simulink model "plot_dynamic_3Drobot"  (R2021a)
settings: Solver=VariableStepAuto  StartTime=0.0  StopTime=100  FixedStep=10e-3  RelTol=1e-3  AbsTol=1e-3  EnableMultiTasking=on
undefined symbols (not defined in the file): C, H, L, L1, L2, L3, X, Y, Z
libraries: sm_lib x38, roblocks x20, nesl_utility x13, simulink x1
settings Model: Creator=Usuário  LastModifiedBy=Usuário
settings SolverCC: AutoScaleAbsTol=off  AlgebraicLoopSolver=TrustRegion
settings DataIOCC: LimitDataPoints=on  MaxDataPoints=10000
settings OptimizationCC: LifeSpan=inf
settings DebuggingCC: AllowSymbolicDim=off  SFUnexpectedBacktrackingDiag=warning  SFNoUnconditionalDefaultTransitionDiag=warning  SFExecutionAtInitializationDiag=none  SFMachineParentedDataDiag=warning  ArithmeticOperatorsInVariantConditions=warning
settings SFSimCC: SimUseLocalCustomCode=off  CustomCodeUndefinedFunction=UseInterfaceOnly
settings RTWCC: RTWUseLocalCustomCode=off
settings CodeAppCC: StateflowObjectComments=on
settings GRTTargetCC: TargetLangStandard=C89/C90 (ANSI)
settings ConfigComp: CovMetricSettings=dw  CovSaveCumulativeToWorkspaceVar=on  CovSaveSingleToWorkspaceVar=on  CovExternalEMLEnable=off  CovSFcnEnable=off
settings SimscapeCC: SimscapeLogType=all  SimscapeLogSimulationStatistics=on  SimscapeLogDataHistory=10000

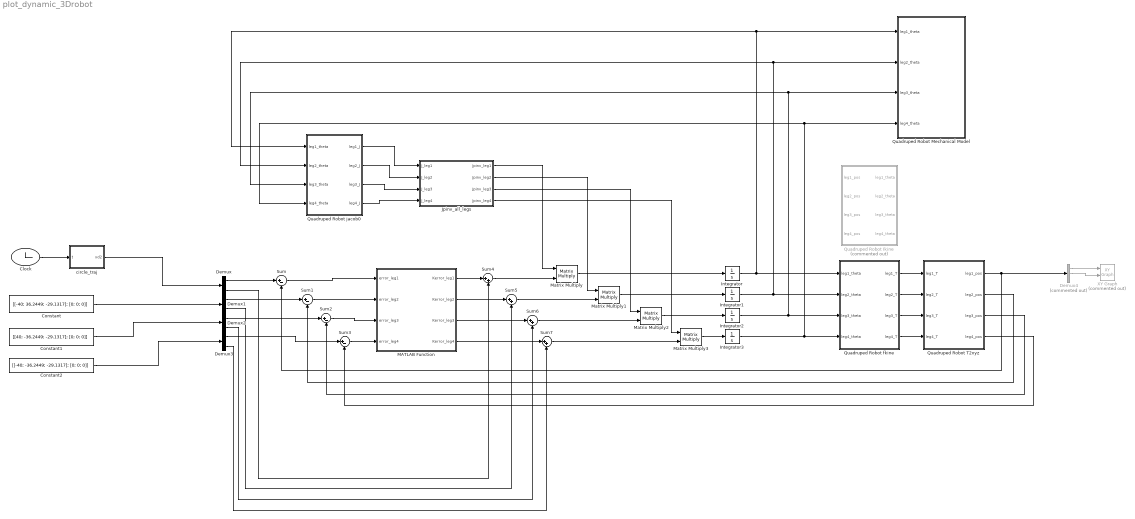
== system plot_dynamic_3Drobot ==
  Clock : Clock
  Constant : Constant  Value=[[-40; 36.2449; -29.1317]; [0; 0; 0]]
  Constant1 : Constant  Value=[[40; -36.2449; -29.1317]; [0; 0; 0]]
  Constant2 : Constant  Value=[[-40; -36.2449; -29.1317]; [0; 0; 0]]
  Demux{,1..3} (4 alike) : Demux  Outputs=2
  Demux4 : Demux  Commented=on  Outputs=3
  Integrator{,1..3} (4 alike) : Integrator
  Jpinv_all_legs : MATLAB Function  TreatAsAtomicUnit=on
  MATLAB Function : MATLAB Function  TreatAsAtomicUnit=on
  Matrix Multiply{,1..3} (4 alike) : Product  Multiplication=Matrix(*)
  Quadruped Robot Ikine : Subsystem  Commented=on
  Quadruped Robot Mechanical Model : Subsystem
  Quadruped Robot T2xyz : Subsystem
  Quadruped Robot fkine : Subsystem
  Quadruped Robot jacob0 : Subsystem
  Sum{,1..3} (4 alike) : Sum  Inputs=|+-
  Sum{4..7} (4 alike) : Sum  Inputs=|++
  XY Graph : simulink/Sinks/XY Graph  Commented=on  xmin=-100  xmax=100  ymin=-100  ymax=100  st=-1
  circle_traj : MATLAB Function  TreatAsAtomicUnit=on
  wires:
  Constant/1 -> Demux1/1
  Constant1/1 -> Demux2/1
  circle_traj/1(xd2) -> Demux/1
  Constant2/1 -> Demux3/1
  Clock/1 -> circle_traj/1(t)
  Quadruped Robot jacob0/1(leg1_J) -> Jpinv_all_legs/1(J_leg1)
  Quadruped Robot jacob0/2(leg2_J) -> Jpinv_all_legs/2(J_leg2)
  Quadruped Robot jacob0/3(leg3_J) -> Jpinv_all_legs/3(J_leg3)
  Quadruped Robot jacob0/4(leg4_J) -> Jpinv_all_legs/4(J_leg4)
  Demux/1 -> Sum/1
  Demux1/1 -> Sum1/1
  Demux2/1 -> Sum2/1
  Demux3/1 -> Sum3/1
  Sum/1 -> MATLAB Function/1(error_leg1)
  Sum1/1 -> MATLAB Function/2(error_leg2)
  Sum2/1 -> MATLAB Function/3(error_leg3)
  Sum3/1 -> MATLAB Function/4(error_leg4)
  MATLAB Function/1(Kerror_leg1) -> Sum4/1
  MATLAB Function/2(Kerror_leg2) -> Sum5/1
  MATLAB Function/3(Kerror_leg3) -> Sum6/1
  MATLAB Function/4(Kerror_leg4) -> Sum7/1
  Demux/2 -> Sum4/2
  Demux1/2 -> Sum5/2
  Demux2/2 -> Sum6/2
  Demux3/2 -> Sum7/2
  Sum4/1 -> Matrix Multiply/2
  Sum5/1 -> Matrix Multiply1/2
  Sum6/1 -> Matrix Multiply2/2
  Sum7/1 -> Matrix Multiply3/2
  Jpinv_all_legs/1(Jpinv_leg1) -> Matrix Multiply/1
  Jpinv_all_legs/2(Jpinv_leg2) -> Matrix Multiply1/1
  Jpinv_all_legs/3(Jpinv_leg3) -> Matrix Multiply2/1
  Jpinv_all_legs/4(Jpinv_leg4) -> Matrix Multiply3/1
  Matrix Multiply/1 -> Integrator/1
  Matrix Multiply1/1 -> Integrator1/1
  Matrix Multiply2/1 -> Integrator2/1
  Matrix Multiply3/1 -> Integrator3/1
  Integrator/1 -> Quadruped Robot fkine/1(leg1_theta), Quadruped Robot jacob0/1(leg1_theta), Quadruped Robot Mechanical Model/1(leg1_theta)
  Integrator1/1 -> Quadruped Robot fkine/2(leg2_theta), Quadruped Robot Mechanical Model/2(leg2_theta), Quadruped Robot jacob0/2(leg2_theta)
  Integrator2/1 -> Quadruped Robot fkine/3(leg3_theta), Quadruped Robot Mechanical Model/3(leg3_theta), Quadruped Robot jacob0/3(leg3_theta)
  Integrator3/1 -> Quadruped Robot fkine/4(leg4_theta), Quadruped Robot Mechanical Model/4(leg4_theta), Quadruped Robot jacob0/4(leg4_theta)
  Quadruped Robot fkine/1(leg1_T) -> Quadruped Robot T2xyz/1(leg1_T)
  Quadruped Robot fkine/2(leg2_T) -> Quadruped Robot T2xyz/2(leg2_T)
  Quadruped Robot fkine/3(leg3_T) -> Quadruped Robot T2xyz/3(leg3_T)
  Quadruped Robot fkine/4(leg4_T) -> Quadruped Robot T2xyz/4(leg4_T)
  Quadruped Robot T2xyz/1(leg1_pos) -> Demux4/1, Sum/2
  Quadruped Robot T2xyz/2(leg2_pos) -> Sum1/2
  Quadruped Robot T2xyz/3(leg3_pos) -> Sum2/2
  Quadruped Robot T2xyz/4(leg4_pos) -> Sum3/2
  Demux4/1 -> XY Graph/1
  Demux4/2 -> XY Graph/2

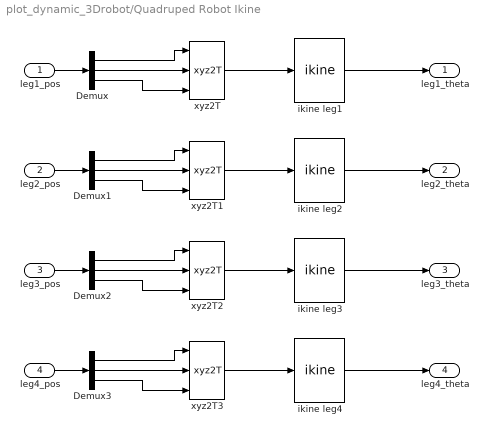
== system plot_dynamic_3Drobot/Quadruped Robot Ikine ==
  leg1_pos : Inport
  leg2_pos : Inport  Port=2
  leg3_pos : Inport  Port=3
  leg4_pos : Inport  Port=4
  Demux{,1..3} (4 alike) : Demux  Outputs=3
  ikine leg1 : roblocks/Arm/ikine  robot=leg1  q0=[0, 0, 0]  M=[1 1 1 0 0 0]  pinv=off  options={'ilimit', 10e4}
      link override ikine: MATLABFcn=robot.ikine(u, 'q0', q0, 'mask', M, opt{:})
  ikine leg2 : roblocks/Arm/ikine  robot=leg2  q0=[0, 0, 0]  M=[1 1 1 0 0 0]  pinv=off  options={'ilimit', 10e4}
      link override ikine: MATLABFcn=robot.ikine(u, 'q0', q0, 'mask', M, opt{:})
  ikine leg3 : roblocks/Arm/ikine  robot=leg3  q0=[0, 0, 0]  M=[1 1 1 0 0 0]  pinv=off  options={'ilimit', 10e4}
      link override ikine: MATLABFcn=robot.ikine(u, 'q0', q0, 'mask', M, opt{:})
  ikine leg4 : roblocks/Arm/ikine  robot=leg4  q0=[0, 0, 0]  M=[1 1 1 0 0 0]  pinv=off  options={'ilimit', 10e4}
      link override ikine: MATLABFcn=robot.ikine(u, 'q0', q0, 'mask', M, opt{:})
  xyz2T{,1..3} (4 alike) : roblocks/Toolbox/xyz2T
  leg1_theta : Outport
  leg2_theta : Outport  Port=2
  leg3_theta : Outport  Port=3
  leg4_theta : Outport  Port=4
  wires:
  xyz2T/1 -> ikine leg1/1
  leg1_pos/1 -> Demux/1
  Demux/1 -> xyz2T/1
  Demux/2 -> xyz2T/2
  Demux/3 -> xyz2T/3
  Demux1/2 -> xyz2T1/2
  Demux1/3 -> xyz2T1/3
  Demux1/1 -> xyz2T1/1
  leg2_pos/1 -> Demux1/1
  xyz2T1/1 -> ikine leg2/1
  Demux2/2 -> xyz2T2/2
  Demux2/3 -> xyz2T2/3
  Demux2/1 -> xyz2T2/1
  leg3_pos/1 -> Demux2/1
  xyz2T2/1 -> ikine leg3/1
  Demux3/2 -> xyz2T3/2
  Demux3/3 -> xyz2T3/3
  Demux3/1 -> xyz2T3/1
  leg4_pos/1 -> Demux3/1
  xyz2T3/1 -> ikine leg4/1
  ikine leg1/1 -> leg1_theta/1
  ikine leg2/1 -> leg2_theta/1
  ikine leg3/1 -> leg3_theta/1
  ikine leg4/1 -> leg4_theta/1

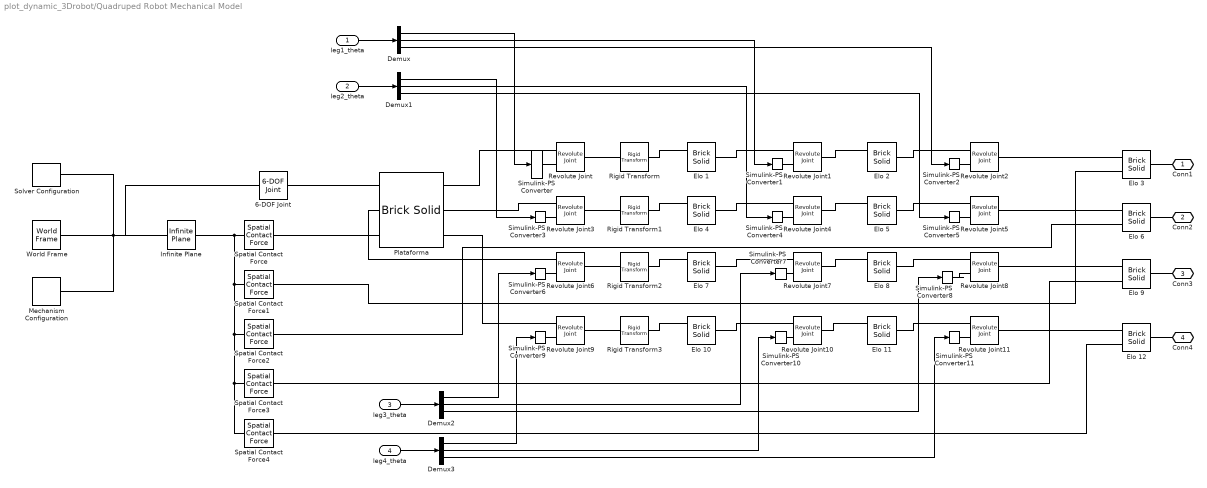
== system plot_dynamic_3Drobot/Quadruped Robot Mechanical Model ==
  leg1_theta : Inport
  leg2_theta : Inport  Port=2
  leg3_theta : Inport  Port=3
  leg4_theta : Inport  Port=4
  6-DOF Joint : sm_lib/Joints/6-DOF Joint  JointMode=Normal  SenseConstraintForce=off  SenseConstraintForceX=off  SenseConstraintForceY=off  SenseConstraintForceZ=off  SenseConstraintTorque=off  SenseConstraintTorqueX=off  SenseConstraintTorqueY=off  SenseConstraintTorqueZ=off  SenseTotalForce=off  SenseTotalForceX=off  SenseTotalForceY=off  SenseTotalForceZ=off  SenseTotalTorque=off  SenseTotalTorqueX=off  SenseTotalTorqueY=off  SenseTotalTorqueZ=off  CompositeWrenchDir=FollowerOnBase  CompositeWrenchFrame=BaseFrame  PxEquilibriumPosition=0  PxEquilibriumPositionUnits=m  PxSpringStiffness=0  PxSpringStiffnessUnits=N/m  PxDampingCoefficient=0  PxDampingCoefficientUnits=N/(m/s)  PxTorqueActuationMode=NoTorque  PxMotionActuationMode=ComputedMotion  PxSensePosition=off  PxSenseVelocity=off  PxSenseAcceleration=off  PxSenseTorqueForce=off  PxSenseLowerLimitTorqueForce=off  PxSenseUpperLimitTorqueForce=off  PxLowerLimitSpecify=off  PxLowerLimitBound=-1  PxLowerLimitBoundUnits=m  PxLowerLimitStiffness=1e6  PxLowerLimitStiffnessUnits=N/m  PxLowerLimitDamping=1e3  PxLowerLimitDampingUnits=N/(m/s)  PxLowerLimitTransitionRegionWidth=1e-4  PxLowerLimitTransitionRegionWidthUnits=m  PxUpperLimitSpecify=off  PxUpperLimitBound=1  PxUpperLimitBoundUnits=m  PxUpperLimitStiffness=1e6  PxUpperLimitStiffnessUnits=N/m  PxUpperLimitDamping=1e3  PxUpperLimitDampingUnits=N/(m/s)  PxUpperLimitTransitionRegionWidth=1e-4  PxUpperLimitTransitionRegionWidthUnits=m  PxPositionTargetSpecify=off  PxPositionTargetPriority=High  PxPositionTargetValue=0  PxPositionTargetValueUnits=m  PxVelocityTargetSpecify=off  PxVelocityTargetPriority=High  PxVelocityTargetValue=0  PxVelocityTargetValueUnits=m/s  PyEquilibriumPosition=0  PyEquilibriumPositionUnits=m  PySpringStiffness=0  PySpringStiffnessUnits=N/m  PyDampingCoefficient=0  PyDampingCoefficientUnits=N/(m/s)  PyTorqueActuationMode=NoTorque  PyMotionActuationMode=ComputedMotion  PySensePosition=off  PySenseVelocity=off  PySenseAcceleration=off  PySenseTorqueForce=off  PySenseLowerLimitTorqueForce=off  PySenseUpperLimitTorqueForce=off  PyLowerLimitSpecify=off  PyLowerLimitBound=-1  PyLowerLimitBoundUnits=m  PyLowerLimitStiffness=1e6  PyLowerLimitStiffnessUnits=N/m  PyLowerLimitDamping=1e3  PyLowerLimitDampingUnits=N/(m/s)  PyLowerLimitTransitionRegionWidth=1e-4  PyLowerLimitTransitionRegionWidthUnits=m  PyUpperLimitSpecify=off  PyUpperLimitBound=1  PyUpperLimitBoundUnits=m  PyUpperLimitStiffness=1e6  PyUpperLimitStiffnessUnits=N/m  PyUpperLimitDamping=1e3  PyUpperLimitDampingUnits=N/(m/s)  PyUpperLimitTransitionRegionWidth=1e-4  PyUpperLimitTransitionRegionWidthUnits=m  PyPositionTargetSpecify=off  PyPositionTargetPriority=High  PyPositionTargetValue=0  PyPositionTargetValueUnits=m  PyVelocityTargetSpecify=off  PyVelocityTargetPriority=High  PyVelocityTargetValue=0  PyVelocityTargetValueUnits=m/s  PzEquilibriumPosition=0  PzEquilibriumPositionUnits=m  PzSpringStiffness=0  PzSpringStiffnessUnits=N/m  PzDampingCoefficient=0  PzDampingCoefficientUnits=N/(m/s)  PzTorqueActuationMode=NoTorque  PzMotionActuationMode=ComputedMotion  PzSensePosition=off  PzSenseVelocity=off  PzSenseAcceleration=off  PzSenseTorqueForce=off  PzSenseLowerLimitTorqueForce=off  PzSenseUpperLimitTorqueForce=off  PzLowerLimitSpecify=off  PzLowerLimitBound=-1  PzLowerLimitBoundUnits=m  PzLowerLimitStiffness=1e6  PzLowerLimitStiffnessUnits=N/m  PzLowerLimitDamping=1e3  PzLowerLimitDampingUnits=N/(m/s)  PzLowerLimitTransitionRegionWidth=1e-4  PzLowerLimitTransitionRegionWidthUnits=m  PzUpperLimitSpecify=off  PzUpperLimitBound=1  PzUpperLimitBoundUnits=m  PzUpperLimitStiffness=1e6  PzUpperLimitStiffnessUnits=N/m  PzUpperLimitDamping=1e3  PzUpperLimitDampingUnits=N/(m/s)  PzUpperLimitTransitionRegionWidth=1e-4  PzUpperLimitTransitionRegionWidthUnits=m  PzPositionTargetSpecify=on  PzPositionTargetPriority=High  PzPositionTargetValue=0.5  PzPositionTargetValueUnits=m  PzVelocityTargetSpecify=off  PzVelocityTargetPriority=High  PzVelocityTargetValue=0  PzVelocityTargetValueUnits=m/s  SphDefPosRotationMethod=None  SphDefPosRotationAngleUnits=deg  SphDefPosRotationStandardAxis=+Z  SphDefPosRotationAngle=0.0  SphDefPosRotationArbitraryAxis=[0 0 1]  SphDefPosFollAlignAxisA=+X  SphDefPosBaseAlignAxisA=+Y  SphDefPosFollAlignAxisB=+Y  SphDefPosBaseAlignAxisB=+Z  SphDefPosRotationSequenceAxes=FollowerAxes  SphDefPosRotationSequence=XYX  SphDefPosRotationSequenceAngles=[0 0 0]  SphDefPosRotationSequenceAnglesUnits=deg  SphDefPosRotationMatrix=[1 0 0; 0 1 0; 0 0 1]  SphEqPosRotationMethod=None  SphEqPosRotationAngleUnits=deg  SphEqPosRotationStandardAxis=+Z  SphEqPosRotationAngle=0.0  SphEqPosRotationArbitraryAxis=[0 0 1]  SphEqPosFollAlignAxisA=+X  SphEqPosBaseAlignAxisA=+Y  SphEqPosFollAlignAxisB=+Y  SphEqPosBaseAlignAxisB=+Z  SphEqPosRotationSequenceAxes=FollowerAxes  SphEqPosRotationSequence=XYX  SphEqPosRotationSequenceAngles=[0 0 0]  SphEqPosRotationSequenceAnglesUnits=deg  SphEqPosRotationMatrix=[1 0 0; 0 1 0; 0 0 1]  SphSpringStiffness=0  SphSpringStiffnessUnits=N*m/deg  SphDampingCoefficient=0  SphDampingCoefficientUnits=N*m/(deg/s)  SphActuateTorqueX=off  SphActuateTorqueY=off  SphActuateTorqueZ=off  SphActuateTorque=off  SphTorqueActuationMode=NoTorque  SphMotionActuationMode=ComputedMotion  SphActuationFrame=BaseFrame  SphSensePosition=off  SphSenseVelocityX=off  SphSenseVelocityY=off  SphSenseVelocityZ=off  SphSenseVelocity=off  SphSenseAccelerationX=off  SphSenseAccelerationY=off  SphSenseAccelerationZ=off  SphSenseAcceleration=off  SphSenseTorqueX=off  SphSenseTorqueY=off  SphSenseTorqueZ=off  SphSenseTorqueForce=off  SphSenseLowerLimitTorqueMag=off  SphSenseUpperLimitTorqueMag=off  SphSensingFrame=BaseFrame  SphLowerLimitSpecify=off  SphLowerLimitBound=15  SphLowerLimitBoundUnits=deg  SphLowerLimitStiffness=1e4  SphLowerLimitStiffnessUnits=N*m/deg  SphLowerLimitDamping=10  SphLowerLimitDampingUnits=N*m/(deg/s)  SphLowerLimitTransitionRegionWidth=0.1  SphLowerLimitTransitionRegionWidthUnits=deg  SphUpperLimitSpecify=off  SphUpperLimitBound=45  SphUpperLimitBoundUnits=deg  SphUpperLimitStiffness=1e4  SphUpperLimitStiffnessUnits=N*m/deg  SphUpperLimitDamping=10  SphUpperLimitDampingUnits=N*m/(deg/s)  SphUpperLimitTransitionRegionWidth=0.1  SphUpperLimitTransitionRegionWidthUnits=deg  SphPositionTargetRotationMethod=None  SphPositionTargetRotationAngleUnits=deg  SphPositionTargetRotationStandardAxis=+Z  SphPositionTargetRotationAngle=0.0  SphPositionTargetRotationArbitraryAxis=[0 0 1]  SphPositionTargetFollAlignAxisA=+X  SphPositionTargetBaseAlignAxisA=+Y  SphPositionTargetFollAlignAxisB=+Y  SphPositionTargetBaseAlignAxisB=+Z  SphPositionTargetRotationSequenceAxes=FollowerAxes  SphPositionTargetRotationSequence=XYX  SphPositionTargetRotationSequenceAngles=[0 0 0]  SphPositionTargetRotationSequenceAnglesUnits=deg  SphPositionTargetRotationMatrix=[1 0 0; 0 1 0; 0 0 1]  SphPositionTargetSpecify=off  SphPositionTargetPriority=High  SphVelocityTargetValue=[0 0 0]  SphVelocityTargetValueUnits=deg/s  SphVelocityTargetSpecify=off  SphVelocityTargetPriority=High  SphVelocityTargetInFollowerFrame=on
  Demux{,1..3} (4 alike) : Demux  Outputs=3
  Elo {1,4,7,10} (4 alike) : sm_lib/Body Elements/Brick Solid  GraphicAmbientColor=[0.15 0.15 0.15 1.0]  BasedOnType=Density  BrickDimensions=[L1 H H]  BrickDimensionUnits=cm  CenterOfMass=[0 0 0]  CenterOfMassUnits=m  GraphicDiffuseColor=[1.0 0.6 0.4]  Density=1000  DensityUnits=kg/m^3  DoExposeReferenceFrame=off  GraphicEmissiveColor=[0.0 0.0 0.0 1.0]  ExportEntireGeometry=on  SerializedFrames=<Frames><Frame><Id>Frame1</Id><Value><Name>B</Name><Origin><Source>GeometricFeature</Source><FeatureName>-x surface</FeatureName></Origin><PrimaryAxis><DefinedDirection>+Y</DefinedDirection><Source>ReferenceFrame</Source><SourceDirection>+Z</SourceDirection><FeatureName></FeatureName></PrimaryAxis><SecondaryAxis><DefinedDirection>+X</DefinedDirection><Source>ReferenceFrame</Source><SourceDirection>+Y</SourceDirection><FeatureName></FeatureName></SecondaryAxis></Value></Frame><Frame><Id>Frame2</Id><Value><Name>E</Name><Origin><Source>GeometricFeature</Source><FeatureName>+x surface</FeatureName></Origin><PrimaryAxis><DefinedDirection>+Y</DefinedDirection><Source>ReferenceFrame</Source><SourceDirection>+Z</SourceDirection><FeatureName></FeatureName></PrimaryAxis><SecondaryAxis><DefinedDirection>+X</DefinedDirection><Source>ReferenceFrame</Source><SourceDirection>+Y</SourceDirection><FeatureName></FeatureName></SecondaryAxis></Value></Frame></Frames>  MarkerShape=Sphere  MarkerSize=10  GraphicType=FromGeometry  InertiaType=CalculateFromGeometry  Mass=1  MassUnits=kg  MomentsOfInertia=[1 1 1]  MomentsOfInertiaUnits=kg*m^2  GraphicOpacity=1.0  ProductsOfInertia=[0 0 0]  ProductsOfInertiaUnits=kg*m^2  GraphicShininess=75  GraphicSpecularColor=[0.5 0.5 0.5 1.0]  GraphicVisPropType=SimpleVisualProperties
  Elo {2,5,8,11} (4 alike) : sm_lib/Body Elements/Brick Solid  GraphicAmbientColor=[0.15 0.15 0.15 1.0]  BasedOnType=Density  BrickDimensions=[L2 H H]  BrickDimensionUnits=cm  CenterOfMass=[0 0 0]  CenterOfMassUnits=m  GraphicDiffuseColor=[1.0 0.4 1.0]  Density=1000  DensityUnits=kg/m^3  DoExposeReferenceFrame=off  GraphicEmissiveColor=[0.0 0.0 0.0 1.0]  ExportEntireGeometry=on  SerializedFrames=<Frames><Frame><Id>Frame1</Id><Value><Name>B</Name><Origin><Source>GeometricFeature</Source><FeatureName>-x surface</FeatureName></Origin><PrimaryAxis><DefinedDirection>+X</DefinedDirection><Source>ReferenceFrame</Source><SourceDirection>-X</SourceDirection><FeatureName></FeatureName></PrimaryAxis><SecondaryAxis><DefinedDirection>+Y</DefinedDirection><Source>ReferenceFrame</Source><SourceDirection>+Y</SourceDirection><FeatureName></FeatureName></SecondaryAxis></Value></Frame><Frame><Id>Frame2</Id><Value><Name>E</Name><Origin><Source>GeometricFeature</Source><FeatureName>+x surface</FeatureName></Origin><PrimaryAxis><DefinedDirection>+Z</DefinedDirection><Source>ReferenceFrame</Source><SourceDirection>-Z</SourceDirection><FeatureName></FeatureName></PrimaryAxis><SecondaryAxis><DefinedDirection>+X</DefinedDirection><Source>ReferenceFrame</Source><SourceDirection>-X</SourceDirection><FeatureName></FeatureName></SecondaryAxis></Value></Frame></Frames>  MarkerShape=Sphere  MarkerSize=10  GraphicType=FromGeometry  InertiaType=CalculateFromGeometry  Mass=1  MassUnits=kg  MomentsOfInertia=[1 1 1]  MomentsOfInertiaUnits=kg*m^2  GraphicOpacity=1.0  ProductsOfInertia=[0 0 0]  ProductsOfInertiaUnits=kg*m^2  GraphicShininess=75  GraphicSpecularColor=[0.5 0.5 0.5 1.0]  GraphicVisPropType=SimpleVisualProperties
  Elo {3,6,9,12} (4 alike) : sm_lib/Body Elements/Brick Solid  GraphicAmbientColor=[0.15 0.15 0.15 1.0]  BasedOnType=Density  BrickDimensions=[L3 H H]  BrickDimensionUnits=cm  CenterOfMass=[0 0 0]  CenterOfMassUnits=m  GraphicDiffuseColor=[0.4 1.0 0.2]  Density=1000  DensityUnits=kg/m^3  DoExposeReferenceFrame=off  GraphicEmissiveColor=[0.0 0.0 0.0 1.0]  ExportEntireGeometry=on  SerializedFrames=<Frames><Frame><Id>Frame1</Id><Value><Name>B</Name><Origin><Source>GeometricFeature</Source><FeatureName>-x surface</FeatureName></Origin><PrimaryAxis><DefinedDirection>+X</DefinedDirection><Source>ReferenceFrame</Source><SourceDirection>-X</SourceDirection><FeatureName></FeatureName></PrimaryAxis><SecondaryAxis><DefinedDirection>+Y</DefinedDirection><Source>ReferenceFrame</Source><SourceDirection>+Y</SourceDirection><FeatureName></FeatureName></SecondaryAxis></Value></Frame><Frame><Id>Frame2</Id><Value><Name>E</Name><Origin><Source>GeometricFeature</Source><FeatureName>+x surface</FeatureName></Origin><PrimaryAxis><DefinedDirection>+Z</DefinedDirection><Source>ReferenceFrame</Source><SourceDirection>-Z</SourceDirection><FeatureName></FeatureName></PrimaryAxis><SecondaryAxis><DefinedDirection>+X</DefinedDirection><Source>ReferenceFrame</Source><SourceDirection>-X</SourceDirection><FeatureName></FeatureName></SecondaryAxis></Value></Frame></Frames>  MarkerShape=Sphere  MarkerSize=10  GraphicType=FromGeometry  InertiaType=CalculateFromGeometry  Mass=1  MassUnits=kg  MomentsOfInertia=[1 1 1]  MomentsOfInertiaUnits=kg*m^2  GraphicOpacity=1.0  ProductsOfInertia=[0 0 0]  ProductsOfInertiaUnits=kg*m^2  GraphicShininess=75  GraphicSpecularColor=[0.5 0.5 0.5 1.0]  GraphicVisPropType=SimpleVisualProperties
  Infinite Plane : sm_lib/Curves and Surfaces/Infinite Plane  GraphicType=Rectangle  GraphicPlaneWidth=5  GraphicPlaneWidthUnits=m  GraphicPlaneHeight=5  GraphicPlaneHeightUnits=m  GraphicVisPropType=SimpleVisualProperties  GraphicDiffuseColor=[0.1843 0.3686 0.5294]  GraphicOpacity=0.75  GraphicSpecularColor=[0.5 0.5 0.5 1.0]  GraphicAmbientColor=[0.15 0.15 0.15 1.0]  GraphicEmissiveColor=[0.0 0.0 0.0 1.0]  GraphicShininess=75
  Mechanism Configuration : sm_lib/Utilities/Mechanism Configuration  UniformGravity=Constant  GravityVector=[0 0 -9.80665]  GravityVectorUnits=m/s^2  GravityUnits=m/s^2  LinearizationDelta=0.001  JointModeTransitionNonlinearIterations=2
  Plataforma : sm_lib/Body Elements/Brick Solid  GraphicAmbientColor=[0.15 0.15 0.15 1.0]  BasedOnType=Density  BrickDimensions=[C L H]  BrickDimensionUnits=cm  CenterOfMass=[0 0 0]  CenterOfMassUnits=m  GraphicDiffuseColor=[0.0 0.8 0.8]  Density=1000  DensityUnits=kg/m^3  DoExposeReferenceFrame=on  GraphicEmissiveColor=[0.0 0.0 0.0 1.0]  ExportEntireGeometry=on  SerializedFrames=<Frames><Frame><Id>Frame1</Id><Value><Name>leg_1</Name><Origin><Source>GeometricFeature</Source><FeatureName>+x +y curve</FeatureName></Origin><PrimaryAxis><DefinedDirection>+Z</DefinedDirection><Source>ReferenceFrame</Source><SourceDirection>+X</SourceDirection><FeatureName></FeatureName></PrimaryAxis><SecondaryAxis><DefinedDirection>+X</DefinedDirection><Source>ReferenceFrame</Source><SourceDirection>-Z</SourceDirection><FeatureName></FeatureName></SecondaryAxis></Value></Frame><Frame><Id>Frame2</Id><Value><Name>leg_2</Name><Origin><Source>GeometricFeature</Source><FeatureName>-x +y curve</FeatureName></Origin><PrimaryAxis><DefinedDirection>+Z</DefinedDirection><Source>ReferenceFrame</Source><SourceDirection>+X</SourceDirection><FeatureName></FeatureName></PrimaryAxis><SecondaryAxis><DefinedDirection>+X</DefinedDirection><Source>ReferenceFrame</Source><SourceDirection>-Z</SourceDirection><FeatureName></FeatureName></SecondaryAxis></Value></Frame><Frame><Id>Frame3</Id><Value><Name>leg_3</Name><Origin><Source>GeometricFeature</Source><FeatureName>+x -y curve</FeatureName></Origin><PrimaryAxis><DefinedDirection>+Z</DefinedDirection><Source>ReferenceFrame</Source><SourceDirection>+X</SourceDirection><FeatureName></FeatureName></PrimaryAxis><SecondaryAxis><DefinedDirection>+X</DefinedDirection><Source>ReferenceFrame</Source><SourceDirection>-Z</SourceDirection><FeatureName></FeatureName></SecondaryAxis></Value></Frame><Frame><Id>Frame4</Id><Value><Name>leg_4</Name><Origin><Source>GeometricFeature</Source><FeatureName>-x -y curve</FeatureName></Origin><PrimaryAxis><DefinedDirection>+Z</DefinedDirection><Source>ReferenceFrame</Source><SourceDirection>+X</SourceDirection><FeatureName></FeatureName></PrimaryAxis><SecondaryAxis><DefinedDirection>+X</DefinedDirection><Source>ReferenceFrame</Source><SourceDirection>-Z</SourceDirection><FeatureName></FeatureName></SecondaryAxis></Value></Frame></Frames>  MarkerShape=Sphere  MarkerSize=10  GraphicType=FromGeometry  InertiaType=CalculateFromGeometry  Mass=1  MassUnits=kg  MomentsOfInertia=[1 1 1]  MomentsOfInertiaUnits=kg*m^2  GraphicOpacity=1.0  ProductsOfInertia=[0 0 0]  ProductsOfInertiaUnits=kg*m^2  GraphicShininess=75  GraphicSpecularColor=[0.5 0.5 0.5 1.0]  GraphicVisPropType=SimpleVisualProperties
  Revolute Joint{,3,6,9} (4 alike) : sm_lib/Joints/Revolute Joint  JointMode=Normal  SenseConstraintForce=off  SenseConstraintForceX=off  SenseConstraintForceY=off  SenseConstraintForceZ=off  SenseConstraintTorque=off  SenseConstraintTorqueX=off  SenseConstraintTorqueY=off  SenseConstraintTorqueZ=off  SenseTotalForce=off  SenseTotalForceX=off  SenseTotalForceY=off  SenseTotalForceZ=off  SenseTotalTorque=off  SenseTotalTorqueX=off  SenseTotalTorqueY=off  SenseTotalTorqueZ=off  CompositeWrenchDir=FollowerOnBase  CompositeWrenchFrame=BaseFrame  EquilibriumPosition=0  EquilibriumPositionUnits=deg  SpringStiffness=0  SpringStiffnessUnits=N*m/deg  DampingCoefficient=0  DampingCoefficientUnits=N*m/(deg/s)  TorqueActuationMode=ComputedTorque  MotionActuationMode=InputMotion  SensePosition=off  SenseVelocity=off  SenseAcceleration=off  SenseTorqueForce=off  SenseLowerLimitTorqueForce=off  SenseUpperLimitTorqueForce=off  LowerLimitSpecify=on  LowerLimitBound=-30  LowerLimitBoundUnits=deg  LowerLimitStiffness=1e4  LowerLimitStiffnessUnits=N*m/deg  LowerLimitDamping=10  LowerLimitDampingUnits=N*m/(deg/s)  LowerLimitTransitionRegionWidth=0.1  LowerLimitTransitionRegionWidthUnits=deg  UpperLimitSpecify=on  UpperLimitBound=30  UpperLimitBoundUnits=deg  UpperLimitStiffness=1e4  UpperLimitStiffnessUnits=N*m/deg  UpperLimitDamping=10  UpperLimitDampingUnits=N*m/(deg/s)  UpperLimitTransitionRegionWidth=0.1  UpperLimitTransitionRegionWidthUnits=deg  PositionTargetSpecify=off  PositionTargetPriority=High  PositionTargetValue=0  PositionTargetValueUnits=deg  VelocityTargetSpecify=off  VelocityTargetPriority=High  VelocityTargetValue=0  VelocityTargetValueUnits=deg/s
  Revolute Joint{1,4,7,10} (4 alike) : sm_lib/Joints/Revolute Joint  JointMode=Normal  SenseConstraintForce=off  SenseConstraintForceX=off  SenseConstraintForceY=off  SenseConstraintForceZ=off  SenseConstraintTorque=off  SenseConstraintTorqueX=off  SenseConstraintTorqueY=off  SenseConstraintTorqueZ=off  SenseTotalForce=off  SenseTotalForceX=off  SenseTotalForceY=off  SenseTotalForceZ=off  SenseTotalTorque=off  SenseTotalTorqueX=off  SenseTotalTorqueY=off  SenseTotalTorqueZ=off  CompositeWrenchDir=FollowerOnBase  CompositeWrenchFrame=BaseFrame  EquilibriumPosition=0  EquilibriumPositionUnits=deg  SpringStiffness=0  SpringStiffnessUnits=N*m/deg  DampingCoefficient=0  DampingCoefficientUnits=N*m/(deg/s)  TorqueActuationMode=ComputedTorque  MotionActuationMode=InputMotion  SensePosition=off  SenseVelocity=off  SenseAcceleration=off  SenseTorqueForce=off  SenseLowerLimitTorqueForce=off  SenseUpperLimitTorqueForce=off  LowerLimitSpecify=on  LowerLimitBound=-60  LowerLimitBoundUnits=deg  LowerLimitStiffness=1e4  LowerLimitStiffnessUnits=N*m/deg  LowerLimitDamping=10  LowerLimitDampingUnits=N*m/(deg/s)  LowerLimitTransitionRegionWidth=0.1  LowerLimitTransitionRegionWidthUnits=deg  UpperLimitSpecify=on  UpperLimitBound=60  UpperLimitBoundUnits=deg  UpperLimitStiffness=1e4  UpperLimitStiffnessUnits=N*m/deg  UpperLimitDamping=10  UpperLimitDampingUnits=N*m/(deg/s)  UpperLimitTransitionRegionWidth=0.1  UpperLimitTransitionRegionWidthUnits=deg  PositionTargetSpecify=off  PositionTargetPriority=High  PositionTargetValue=0  PositionTargetValueUnits=deg  VelocityTargetSpecify=off  VelocityTargetPriority=High  VelocityTargetValue=0  VelocityTargetValueUnits=deg/s
  Revolute Joint{2,5,8,11} (4 alike) : sm_lib/Joints/Revolute Joint  JointMode=Normal  SenseConstraintForce=off  SenseConstraintForceX=off  SenseConstraintForceY=off  SenseConstraintForceZ=off  SenseConstraintTorque=off  SenseConstraintTorqueX=off  SenseConstraintTorqueY=off  SenseConstraintTorqueZ=off  SenseTotalForce=off  SenseTotalForceX=off  SenseTotalForceY=off  SenseTotalForceZ=off  SenseTotalTorque=off  SenseTotalTorqueX=off  SenseTotalTorqueY=off  SenseTotalTorqueZ=off  CompositeWrenchDir=FollowerOnBase  CompositeWrenchFrame=BaseFrame  EquilibriumPosition=0  EquilibriumPositionUnits=deg  SpringStiffness=0  SpringStiffnessUnits=N*m/deg  DampingCoefficient=0  DampingCoefficientUnits=N*m/(deg/s)  TorqueActuationMode=ComputedTorque  MotionActuationMode=InputMotion  SensePosition=off  SenseVelocity=off  SenseAcceleration=off  SenseTorqueForce=off  SenseLowerLimitTorqueForce=off  SenseUpperLimitTorqueForce=off  LowerLimitSpecify=on  LowerLimitBound=-90  LowerLimitBoundUnits=deg  LowerLimitStiffness=1e4  LowerLimitStiffnessUnits=N*m/deg  LowerLimitDamping=10  LowerLimitDampingUnits=N*m/(deg/s)  LowerLimitTransitionRegionWidth=0.1  LowerLimitTransitionRegionWidthUnits=deg  UpperLimitSpecify=on  UpperLimitBound=0  UpperLimitBoundUnits=deg  UpperLimitStiffness=1e4  UpperLimitStiffnessUnits=N*m/deg  UpperLimitDamping=10  UpperLimitDampingUnits=N*m/(deg/s)  UpperLimitTransitionRegionWidth=0.1  UpperLimitTransitionRegionWidthUnits=deg  PositionTargetSpecify=off  PositionTargetPriority=High  PositionTargetValue=0  PositionTargetValueUnits=deg  VelocityTargetSpecify=off  VelocityTargetPriority=High  VelocityTargetValue=0  VelocityTargetValueUnits=deg/s
  Rigid Transform : sm_lib/Frames and Transforms/Rigid Transform  TranslationMethod=None  TranslationStandardOffset=0  TranslationLengthUnit=m  TranslationStandardAxis=+Z  TranslationCartesianOffset=[0 0 0]  TranslationROffset=0  TranslationROffsetUnits=m  TranslationZOffset=0  TranslationZOffsetUnits=m  TranslationThetaOffset=0  TranslationThetaOffsetUnits=deg  RotationMethod=RotationMatrix  RotationAngleUnits=deg  RotationStandardAxis=+Z  RotationAngle=0.0  RotationArbitraryAxis=[0 0 1]  FollAlignAxisA=+X  BaseAlignAxisA=+Y  FollAlignAxisB=+Y  BaseAlignAxisB=+Z  RotationSequenceAxes=FollowerAxes  RotationSequence=XYX  RotationSequenceAngles=[0 0 0]  RotationSequenceAnglesUnits=deg  RotationMatrix=[-1 0 0; 0 0 1; 0 1 0]
  Rigid Transform1 : sm_lib/Frames and Transforms/Rigid Transform  TranslationMethod=None  TranslationStandardOffset=0  TranslationLengthUnit=m  TranslationStandardAxis=+Z  TranslationCartesianOffset=[0 0 0]  TranslationROffset=0  TranslationROffsetUnits=m  TranslationZOffset=0  TranslationZOffsetUnits=m  TranslationThetaOffset=0  TranslationThetaOffsetUnits=deg  RotationMethod=RotationMatrix  RotationAngleUnits=deg  RotationStandardAxis=+Z  RotationAngle=0.0  RotationArbitraryAxis=[0 0 1]  FollAlignAxisA=+X  BaseAlignAxisA=+Y  FollAlignAxisB=+Y  BaseAlignAxisB=+Z  RotationSequenceAxes=FollowerAxes  RotationSequence=XYX  RotationSequenceAngles=[0 0 0]  RotationSequenceAnglesUnits=deg  RotationMatrix=[-1 0 0; 0 0 1; 0 1 0]
  Rigid Transform2 : sm_lib/Frames and Transforms/Rigid Transform  TranslationMethod=None  TranslationStandardOffset=0  TranslationLengthUnit=m  TranslationStandardAxis=+Z  TranslationCartesianOffset=[0 0 0]  TranslationROffset=0  TranslationROffsetUnits=m  TranslationZOffset=0  TranslationZOffsetUnits=m  TranslationThetaOffset=0  TranslationThetaOffsetUnits=deg  RotationMethod=RotationMatrix  RotationAngleUnits=deg  RotationStandardAxis=+Z  RotationAngle=0.0  RotationArbitraryAxis=[0 0 1]  FollAlignAxisA=+X  BaseAlignAxisA=+Y  FollAlignAxisB=+Y  BaseAlignAxisB=+Z  RotationSequenceAxes=FollowerAxes  RotationSequence=XYX  RotationSequenceAngles=[0 0 0]  RotationSequenceAnglesUnits=deg  RotationMatrix=[-1 0 0; 0 0 -1; 0 -1 0]
  Rigid Transform3 : sm_lib/Frames and Transforms/Rigid Transform  TranslationMethod=None  TranslationStandardOffset=0  TranslationLengthUnit=m  TranslationStandardAxis=+Z  TranslationCartesianOffset=[0 0 0]  TranslationROffset=0  TranslationROffsetUnits=m  TranslationZOffset=0  TranslationZOffsetUnits=m  TranslationThetaOffset=0  TranslationThetaOffsetUnits=deg  RotationMethod=RotationMatrix  RotationAngleUnits=deg  RotationStandardAxis=+Z  RotationAngle=0.0  RotationArbitraryAxis=[0 0 1]  FollAlignAxisA=+X  BaseAlignAxisA=+Y  FollAlignAxisB=+Y  BaseAlignAxisB=+Z  RotationSequenceAxes=FollowerAxes  RotationSequence=XYX  RotationSequenceAngles=[0 0 0]  RotationSequenceAnglesUnits=deg  RotationMatrix=[-1 0 0; 0 0 -1; 0 -1 0]
  Simulink-PS Converter{,1..11} (12 alike) : nesl_utility/Simulink-PS Converter  PhysicalDomain=network_engine_domain  SubClassName=ps_input  LeftPortType=input  RightPortType=output  PseudoPeriodic=off  Frequencies=[]  NoiseDistribution=none  NoiseParameters=[]  Unit=1  AffineConversion=off  FilteringAndDerivatives=filter  SimscapeFilterOrder=2  InputFilterTimeConstant=0.001  UdotUserProvided=0
      settings: SourceProductBaseCode=PW,SS
  Solver Configuration : nesl_utility/Solver Configuration  PhysicalDomain=network_engine_domain  SubClassName=solver  LeftPortType=input  RightPortType=generic  Tones=[]  Harmonics=[]  SimulateNoise=off  Profile=off  UseLocalSampling=off  EnableSwitchedLinearOptims=on  FrequencyDomain=off  UseCCode=off  RelTol=0.001  AbsTol=1e-06  MinStep=1e-09  ToWorkspace=off  RevertToSquareIcSolve=off  NumHomotopyIterations=100  PhasorMode=off  PhasorModeNumHarmonics=1  DoDC=off  ResidualTolerance=1e-09  UseLocalSolver=off  LocalSolverChoice=NE_BACKWARD_EULER_ADVANCER  LocalSolverSampleTime=0.001  DoFixedCost=off  MaxNonlinIter=3  MaxModeIter=2  ComputeImpulses=off  ImpulseIterations=2  LinearAlgebra=Sparse  EquationFormulation=NE_TIME_EF  DelaysMemoryBudget=1024  AutomaticFiltering=on  FilteringTimeConstant=0.001  PartitionStorageMethod=AS_NEEDED  PartitionMemoryBudget=1024  PartitionMethod=FAST
      settings: SourceProductBaseCode=PW,SS
  Spatial Contact Force{,1..4} (5 alike) : sm_lib/Forces and Torques/Spatial Contact Force  CoefficientOfDynamicFriction=0.3  CoefficientOfStaticFriction=0.5  SenseContactBaseRotation=off  SenseContactBaseTranslation=off  NormalDamping=1e3  NormalDampingUnits=N/(m/s)  SenseContactFollowerRotation=off  SenseContactFollowerTranslation=off  SenseContactSignal=off  NormalStiffness=1e6  NormalStiffnessUnits=N/m  FrictionalCriticalVelocity=1e-3  FrictionalCriticalVelocityUnits=m/s  ZeroCrossDetectContactStartAndEnd=off  FrictionType=SmoothStickSlip  SenseFrictionalForceMagnitude=off  SenseNormalForceMagnitude=off  NormalForceType=SmoothSpringDamper  SenseNormalVelocity=off  SenseSeparationDistance=off  SenseTangentialVelocity=off  SenseTangentialVelocityMagnitude=off  NormalTransitionRegionWidth=1e-4  NormalTransitionRegionWidthUnits=m
  World Frame : sm_lib/Frames and Transforms/World Frame
  Conn1 : PMIOPort  Side=Right
  Conn2 : PMIOPort  Port=2  Side=Right
  Conn3 : PMIOPort  Port=3  Side=Right
  Conn4 : PMIOPort  Port=4  Side=Right
  wires:
  Demux2/2 -> Simulink-PS Converter7/1
  Demux2/3 -> Simulink-PS Converter8/1
  Demux3/2 -> Simulink-PS Converter10/1
  Demux/3 -> Simulink-PS Converter2/1
  Demux3/3 -> Simulink-PS Converter11/1
  Demux1/2 -> Simulink-PS Converter4/1
  Demux1/3 -> Simulink-PS Converter5/1
  Demux/1 -> Simulink-PS Converter/1
  Demux2/1 -> Simulink-PS Converter6/1
  Demux/2 -> Simulink-PS Converter1/1
  Demux3/1 -> Simulink-PS Converter9/1
  leg1_theta/1 -> Demux/1
  leg2_theta/1 -> Demux1/1
  Demux1/1 -> Simulink-PS Converter3/1
  leg3_theta/1 -> Demux2/1
  leg4_theta/1 -> Demux3/1
  connections:
  Revolute Joint9/LConn2 -- Simulink-PS Converter9/RConn1
  Revolute Joint8/RConn1 -- Elo 9/LConn1
  Revolute Joint10/LConn1 -- Elo 10/RConn1
  Elo 12/RConn1 -- Conn4/RConn1
  Elo 9/RConn1 -- Conn3/RConn1
  Revolute Joint9/LConn1 -- Plataforma/LConn3
  Simulink-PS Converter/RConn1 -- Revolute Joint/LConn2
  Revolute Joint2/LConn1 -- Elo 2/RConn1
  Revolute Joint6/LConn1 -- Plataforma/RConn2
  Elo 8/LConn1 -- Revolute Joint7/RConn1
  Revolute Joint5/LConn2 -- Simulink-PS Converter5/RConn1
  Elo 11/LConn1 -- Revolute Joint10/RConn1
  Revolute Joint11/LConn2 -- Simulink-PS Converter11/RConn1
  Elo 6/RConn1 -- Conn2/RConn1
  Elo 1/LConn1 -- Rigid Transform/RConn1
  Revolute Joint7/LConn1 -- Elo 7/RConn1
  Revolute Joint5/RConn1 -- Elo 6/LConn1
  Revolute Joint11/LConn1 -- Elo 11/RConn1
  Revolute Joint8/LConn1 -- Elo 8/RConn1
  Rigid Transform/LConn1 -- Revolute Joint/RConn1
  Rigid Transform2/LConn1 -- Revolute Joint6/RConn1
  Revolute Joint3/LConn1 -- Plataforma/LConn2
  Revolute Joint5/LConn1 -- Elo 5/RConn1
  Elo 7/LConn1 -- Rigid Transform2/RConn1
  Revolute Joint1/LConn2 -- Simulink-PS Converter1/RConn1
  Revolute Joint4/LConn1 -- Elo 4/RConn1
  Revolute Joint11/RConn1 -- Elo 12/LConn1
  Plataforma/LConn1 -- Revolute Joint/LConn1
  Elo 4/LConn1 -- Rigid Transform1/RConn1
  Elo 3/RConn1 -- Conn1/RConn1
  Revolute Joint2/RConn1 -- Elo 3/LConn1
  Revolute Joint10/LConn2 -- Simulink-PS Converter10/RConn1
  Elo 2/LConn1 -- Revolute Joint1/RConn1
  Revolute Joint2/LConn2 -- Simulink-PS Converter2/RConn1
  Revolute Joint1/LConn1 -- Elo 1/RConn1
  Rigid Transform1/LConn1 -- Revolute Joint3/RConn1
  Rigid Transform3/LConn1 -- Revolute Joint9/RConn1
  Elo 10/LConn1 -- Rigid Transform3/RConn1
  Revolute Joint4/LConn2 -- Simulink-PS Converter4/RConn1
  Elo 5/LConn1 -- Revolute Joint4/RConn1
  Revolute Joint6/LConn2 -- Simulink-PS Converter6/RConn1
  Revolute Joint3/LConn2 -- Simulink-PS Converter3/RConn1
  Revolute Joint7/LConn2 -- Simulink-PS Converter7/RConn1
  Simulink-PS Converter8/RConn1 -- Revolute Joint8/LConn2
  World Frame/RConn1 -- Infinite Plane/LConn1 -- 6-DOF Joint/LConn1 -- Mechanism Configuration/RConn1 -- Solver Configuration/RConn1
  Infinite Plane/RConn1 -- Spatial Contact Force4/LConn1 -- Spatial Contact Force3/LConn1 -- Spatial Contact Force2/LConn1 -- Spatial Contact Force1/LConn1 -- Spatial Contact Force/LConn1
  Spatial Contact Force/RConn1 -- Plataforma/RConn3
  Plataforma/RConn1 -- 6-DOF Joint/RConn1
  Spatial Contact Force1/RConn1 -- Elo 3/LConn2
  Spatial Contact Force2/RConn1 -- Elo 6/LConn2
  Spatial Contact Force3/RConn1 -- Elo 9/LConn2
  Spatial Contact Force4/RConn1 -- Elo 12/LConn2

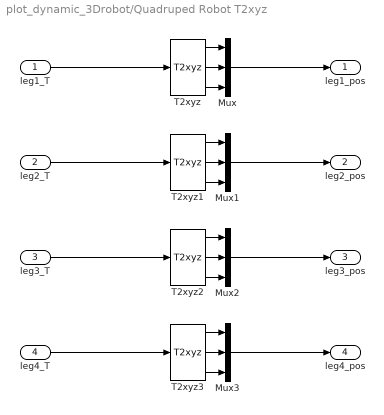
== system plot_dynamic_3Drobot/Quadruped Robot T2xyz ==
  leg1_T : Inport
  leg2_T : Inport  Port=2
  leg3_T : Inport  Port=3
  leg4_T : Inport  Port=4
  Mux{,1..3} (4 alike) : Mux  Inputs=3
  T2xyz{,1..3} (4 alike) : roblocks/Toolbox/T2xyz
  leg1_pos : Outport
  leg2_pos : Outport  Port=2
  leg3_pos : Outport  Port=3
  leg4_pos : Outport  Port=4
  wires:
  leg2_T/1 -> T2xyz1/1
  Mux/1 -> leg1_pos/1
  leg1_T/1 -> T2xyz/1
  Mux1/1 -> leg2_pos/1
  Mux2/1 -> leg3_pos/1
  leg4_T/1 -> T2xyz3/1
  leg3_T/1 -> T2xyz2/1
  Mux3/1 -> leg4_pos/1
  T2xyz/1 -> Mux/1
  T2xyz/2 -> Mux/2
  T2xyz/3 -> Mux/3
  T2xyz1/1 -> Mux1/1
  T2xyz1/2 -> Mux1/2
  T2xyz1/3 -> Mux1/3
  T2xyz2/1 -> Mux2/1
  T2xyz2/2 -> Mux2/2
  T2xyz2/3 -> Mux2/3
  T2xyz3/3 -> Mux3/3
  T2xyz3/1 -> Mux3/1
  T2xyz3/2 -> Mux3/2

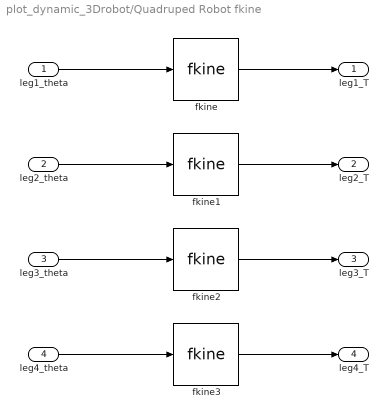
== system plot_dynamic_3Drobot/Quadruped Robot fkine ==
  leg1_theta : Inport
  leg2_theta : Inport  Port=2
  leg3_theta : Inport  Port=3
  leg4_theta : Inport  Port=4
  fkine : roblocks/Arm/fkine  robot=leg1
  fkine1 : roblocks/Arm/fkine  robot=leg2
  fkine2 : roblocks/Arm/fkine  robot=leg3
  fkine3 : roblocks/Arm/fkine  robot=leg4
  leg1_T : Outport
  leg2_T : Outport  Port=2
  leg3_T : Outport  Port=3
  leg4_T : Outport  Port=4
  wires:
  leg2_theta/1 -> fkine1/1
  fkine/1 -> leg1_T/1
  leg1_theta/1 -> fkine/1
  fkine1/1 -> leg2_T/1
  fkine2/1 -> leg3_T/1
  leg4_theta/1 -> fkine3/1
  leg3_theta/1 -> fkine2/1
  fkine3/1 -> leg4_T/1

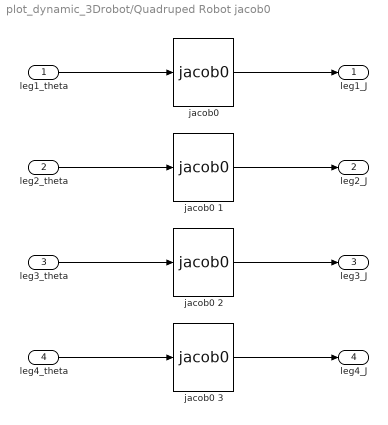
== system plot_dynamic_3Drobot/Quadruped Robot jacob0 ==
  leg1_theta : Inport
  leg2_theta : Inport  Port=2
  leg3_theta : Inport  Port=3
  leg4_theta : Inport  Port=4
  "jacob0 " : roblocks/Arm/jacob0   robot=leg1
  jacob0 1 : roblocks/Arm/jacob0   robot=leg2
  jacob0 2 : roblocks/Arm/jacob0   robot=leg3
  jacob0 3 : roblocks/Arm/jacob0   robot=leg4
  leg1_J : Outport
  leg2_J : Outport  Port=2
  leg3_J : Outport  Port=3
  leg4_J : Outport  Port=4
  wires:
  leg2_theta/1 -> jacob0 1/1
  "jacob0 "/1 -> leg1_J/1
  leg1_theta/1 -> "jacob0 "/1
  jacob0 1/1 -> leg2_J/1
  jacob0 2/1 -> leg3_J/1
  leg4_theta/1 -> jacob0 3/1
  leg3_theta/1 -> jacob0 2/1
  jacob0 3/1 -> leg4_J/1

== matlab function plot_dynamic_3Drobot/Jpinv_all_legs ==
  data: J_leg1 input; Jpinv_leg1 output; J_leg2 input; J_leg3 input; J_leg4 input; Jpinv_leg2 output; Jpinv_leg3 output; Jpinv_leg4 output
function [Jpinv_leg1, Jpinv_leg2, Jpinv_leg3, Jpinv_leg4] = Jpinv_all_legs(J_leg1, J_leg2, J_leg3, J_leg4)

%revisar esse slice do jacobiano
Jpinv_leg1 = pinv(J_leg1(1:3,1:3));
Jpinv_leg2 = pinv(J_leg2(1:3,1:3));
Jpinv_leg3 = pinv(J_leg3(1:3,1:3));
Jpinv_leg4 = pinv(J_leg4(1:3,1:3));

== matlab function plot_dynamic_3Drobot/circle_traj ==
  data: t input; xd2 output
function xd2 = circle_traj(t)
wn = pi/2;          % Frequência angular (rad/s)
r = 15;            % Raio da circunferência (m)
x0 = [40; 25; -17]; % Centro da circunferência no plano X-Z

% Trajetória no plano X-Y
xd = [x0(1) + r*cos(wn*t);
      x0(2) + r*sin(wn*t);
      x0(3)];

% Velocidade (derivada de xd em relação ao tempo)
xddot = [-r*wn*sin(wn*t);
          r*wn*cos(wn*t);
          0];

xd2 = [xd; xddot];

== matlab function plot_dynamic_3Drobot/MATLAB Function ==
  data: error_leg1 input; Kerror_leg1 output; error_leg2 input; error_leg3 input; error_leg4 input; Kerror_leg2 output; Kerror_leg3 output; Kerror_leg4 output
function [Kerror_leg1, Kerror_leg2, Kerror_leg3, Kerror_leg4] = gain_all_legs(error_leg1, error_leg2, error_leg3, error_leg4)

% revisar o valor desse ganho
K_leg1 = 1;
K_leg2 = 1;
K_leg3 = 1;
K_leg4 = 1;

Kerror_leg1 = K_leg1 * error_leg1;
Kerror_leg2 = K_leg2 * error_leg2;
Kerror_leg3 = K_leg3 * error_leg3;
Kerror_leg4 = K_leg4 * error_leg4;
